simulink model "PPT_sim"  (R2023b)
settings: Solver=VariableStepAuto  StartTime=0.0  StopTime=Tstop  FixedStep=1e-9  RelTol=1e-3
values from neighbouring files (symbols this model uses):
  F_constant = (0.5 * Lpe)    (= 1.88495559215e-06)    [Electrical_model.m]
  Lpe = (mu_o/(4*pi))*log(r_o/r_i)    [Electrical_model.m]
  Re = 5e-3    (= 0.005)    [Electrical_model.m]
  Rp = 15e-3    (= 0.015)    [Electrical_model.m]
  Rpe = 5e-3    (= 0.005)    [Electrical_model.m]
libraries: fl_lib x8, nesl_utility x6, ee_lib x3
settings Model: Creator=georges  LastModifiedBy=georges

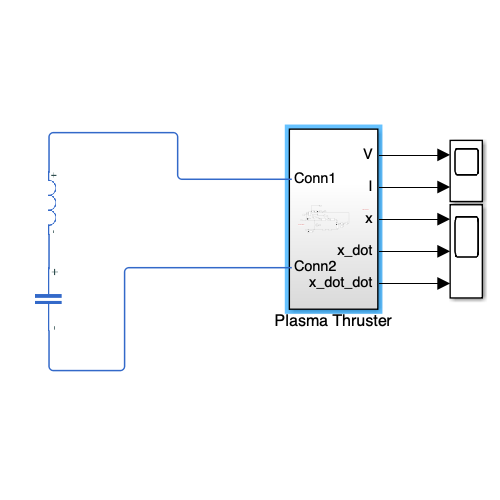
[thumbnail: Simulink's stored preview of the top-level diagram]
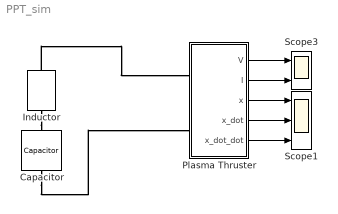
== system PPT_sim ==
  Capacitor : fl_lib/Electrical/Electrical Elements/Capacitor  c=C F  r=0 Ohm  g=0 1/Ohm  i_specify=off  i_priority=None  i=0 A  i_nominal_specify=off  i_nominal_unit=A  i_nominal_value=1  v_specify=off  v_priority=None  v=0 V  v_nominal_specify=off  v_nominal_unit=V  v_nominal_value=1  vc_specify=on  vc_priority=High  vc=V_o V  vc_nominal_specify=off  vc_nominal_unit=V  vc_nominal_value=1
  Inductor : fl_lib/Electrical/Electrical Elements/Inductor  l=C_l H  r=C_r Ohm  g=1e-9 1/Ohm  i_specify=off  i_priority=None  i=0 A  i_nominal_specify=off  i_nominal_unit=A  i_nominal_value=1  v_specify=off  v_priority=None  v=0 V  v_nominal_specify=off  v_nominal_unit=V  v_nominal_value=1  i_L_specify=off  i_L_priority=High  i_L=0 A  i_L_nominal_specify=off  i_L_nominal_unit=A  i_L_nominal_value=1
  Plasma Thruster : Subsystem
  Scope1 : Scope  NumInputPorts=3
  Scope3 : Scope  NumInputPorts=2
  wires:
  Plasma Thruster/1(V) -> Scope3/1
  Plasma Thruster/2(I) -> Scope3/2
  Plasma Thruster/3(x) -> Scope1/1
  Plasma Thruster/4(x_dot) -> Scope1/2
  Plasma Thruster/5(x_dot_dot) -> Scope1/3
  connections:
  Inductor/RConn1 -- Capacitor/LConn1
  Inductor/LConn1 -- Plasma Thruster/LConn1
  Capacitor/RConn1 -- Plasma Thruster/LConn2

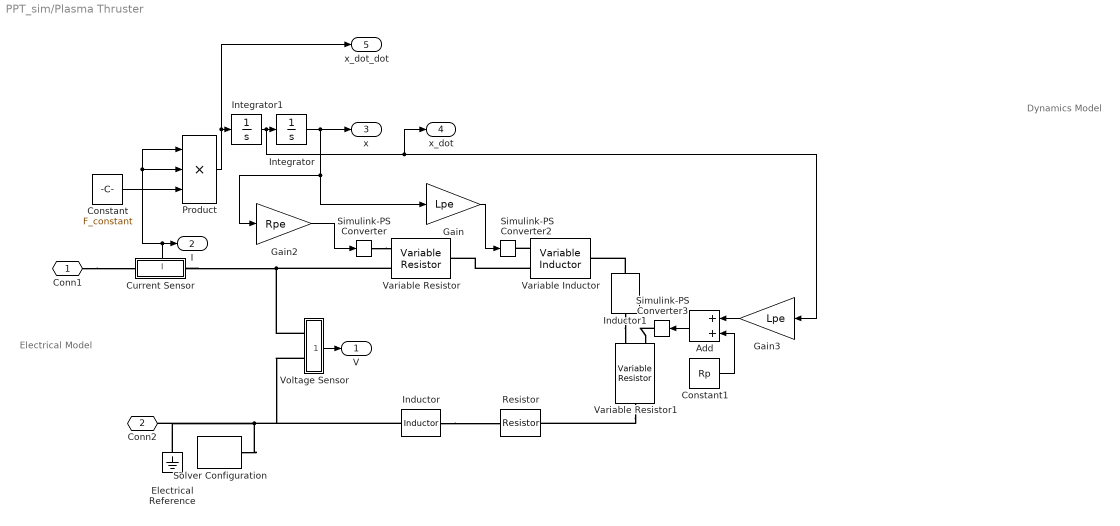
== system PPT_sim/Plasma Thruster ==
  note: Dynamics Model
  note: Electrical Model
  Add : Sum
  Constant : Constant  Value=F_constant
  Constant1 : Constant  Value=Rp
  Current Sensor : Subsystem
      settings: PortSchema="{\"entries\":[{\"content\":{\"sides\":[{\"content\":{\"connectorIds\":[\"LConn1\"]},\"type\":\"ConnectorPlacement.EquallySpacedRectSide\",\"uuid\":\"4e3d035d-d1bd-44cd-bdc3-798a8c03f7f9\"},{\"content\":{\"connectorIds\":[\"RConn1\"],\"side\":\"RIGHT\"},\"type\":\"ConnectorPlacement.EquallySpacedRectSide\",\"uuid\":\"472486ae-4f6c-481a-85ae-821eac2c32db\"},{\"content\":{\"connectorIds\":[\"Out1\"],\"side\":\"TOP\"},\"type\":\"ConnectorPlacement.EquallySpacedRectSide\",\"uuid\":\"f6d4bb52-0012-4c25-b68a-f3fc5d7680d6\"},{\"content\":{\"side\":\"BOTTOM\"},\"type\":\"ConnectorPlacement.EquallySpacedRectSide\",\"uuid\":\"a1fb2eff-50b5-40ce-849c-411f22b22d47\"}]},\"type\":\"ConnectorPlacement.EquallySpacedConnector\",\"uuid\":\"c1379bfe-a6a4-4840-8ba9-3be7ee51b238\"}],\"packageUris\":[\"http://schema.mathworks.com/mf0/Connector/R2020b\"],\"version\":\"1.0\"}"
  Electrical Reference : fl_lib/Electrical/Electrical Elements/Electrical Reference
  Gain : Gain  Gain=Lpe
  Gain2 : Gain  Gain=Rpe
  Gain3 : Gain  Gain=Lpe
  Inductor : ee_lib/Passive/Inductor  l=Le H  enable_L_tol=ee.enum.toleranceApplication.none  L_tol=20  tol_distribution=ee.enum.toleranceDistribution.uniform  nSigma=4  r=0 Ohm  g=0 1/Ohm  enable_operating_limits=ee.enum.enable.no  operating_limit_action=ee.enum.passive.reportOpLim.warn  max_working_current=1 A  power_rating=1 W  enable_faults=ee.enum.enable.no  fault_action=simscape.enum.assert.action.none  lambdaPercent=50  k_faulted=0.9999  turnsShort=ee.enum.passive.inductor.turnsShortOption.no  openCct=ee.enum.enable.no  groundShort=ee.enum.passive.inductor.groundShortOption.no  groundShortG=0 1/Ohm  tau_fault=1e-3 s  fault_trigger=ee.enum.faults.faultTrigger.temporal  t_fault=1 s  max_permissible_voltage=100 V  n_fail_on_voltage=1  max_permissible_current=1 A  t_fail_on_current=1 s  i_L_specify=off  i_L_priority=High  i_L=0 A  i_L_nominal_specify=off  i_L_nominal_unit=A  i_L_nominal_value=1
  Inductor1 : ee_lib/Passive/Inductor  l=Lp H  enable_L_tol=ee.enum.toleranceApplication.none  L_tol=20  tol_distribution=ee.enum.toleranceDistribution.uniform  nSigma=4  r=0 Ohm  g=0 1/Ohm  enable_operating_limits=ee.enum.enable.no  operating_limit_action=ee.enum.passive.reportOpLim.warn  max_working_current=1 A  power_rating=1 W  enable_faults=ee.enum.enable.no  fault_action=simscape.enum.assert.action.none  lambdaPercent=50  k_faulted=0.9999  turnsShort=ee.enum.passive.inductor.turnsShortOption.no  openCct=ee.enum.enable.no  groundShort=ee.enum.passive.inductor.groundShortOption.no  groundShortG=0 1/Ohm  tau_fault=1e-3 s  fault_trigger=ee.enum.faults.faultTrigger.temporal  t_fault=1 s  max_permissible_voltage=100 V  n_fail_on_voltage=1  max_permissible_current=1 A  t_fail_on_current=1 s  i_L_specify=off  i_L_priority=High  i_L=0 A  i_L_nominal_specify=off  i_L_nominal_unit=A  i_L_nominal_value=1
  Integrator : Integrator
  Integrator1 : Integrator
  Product : Product  Inputs=3
  Resistor : fl_lib/Electrical/Electrical Elements/Resistor  R=Re Ohm  i_specify=off  i_priority=None  i=0 A  i_nominal_specify=off  i_nominal_unit=A  i_nominal_value=1  v_specify=off  v_priority=None  v=0 V  v_nominal_specify=off  v_nominal_unit=V  v_nominal_value=1
  Simulink-PS Converter : nesl_utility/Simulink-PS Converter  PhysicalDomain=network_engine_domain  SubClassName=ps_input  LeftPortType=input  RightPortType=output  PseudoPeriodic=off  Frequencies=[]  NoiseDistribution=none  NoiseParameters=[]  Unit=1  AffineConversion=off  FilteringAndDerivatives=provide  SimscapeFilterOrder=1  InputFilterTimeConstant=0.001  UdotUserProvided=0
  Simulink-PS Converter2 : nesl_utility/Simulink-PS Converter  PhysicalDomain=network_engine_domain  SubClassName=ps_input  LeftPortType=input  RightPortType=output  PseudoPeriodic=off  Frequencies=[]  NoiseDistribution=none  NoiseParameters=[]  Unit=1  AffineConversion=off  FilteringAndDerivatives=provide  SimscapeFilterOrder=1  InputFilterTimeConstant=0.001  UdotUserProvided=0
  Simulink-PS Converter3 : nesl_utility/Simulink-PS Converter  PhysicalDomain=network_engine_domain  SubClassName=ps_input  LeftPortType=input  RightPortType=output  PseudoPeriodic=off  Frequencies=[]  NoiseDistribution=none  NoiseParameters=[]  Unit=1  AffineConversion=off  FilteringAndDerivatives=provide  SimscapeFilterOrder=1  InputFilterTimeConstant=0.001  UdotUserProvided=0
  Solver Configuration : nesl_utility/Solver Configuration  PhysicalDomain=network_engine_domain  SubClassName=solver  LeftPortType=input  RightPortType=generic  Tones=[]  Harmonics=[]  SimulateNoise=off  Profile=off  UseLocalSampling=off  EnableSwitchedLinearOptims=on  FrequencyDomain=off  UseCCode=off  RelTol=0.001  AbsTol=0.001  MinStep=1e-09  ToWorkspace=off  RevertToSquareIcSolve=off  NumHomotopyIterations=100  PhasorMode=off  PhasorModeNumHarmonics=1  ConsistencySolver=NEWTON_XTOL_AFTER_FTOL  IndexReductionMethod=DerivativeReplacement  DoDC=off  ResidualTolerance=1e-09  ConsistencyTolSource=GLOBAL  ConsistencyAbsTol=0.001  ConsistencyRelTol=0.001  ConsistencyTolFactor=0.001  UseLocalSolver=off  LocalSolverChoice=NE_BACKWARD_EULER_ADVANCER  ResolveIndetEquations=on  FunctionEvalNumThread=1  LocalSolverSampleTime=0.001  DoFixedCost=off  MaxNonlinIter=3  MaxModeIter=2  ComputeImpulses=off  ImpulseIterations=2  LinearAlgebra=auto  LinearAlgebraNumThread=0  EquationFormulation=NE_TIME_EF  DelaysMemoryBudget=1024  AutomaticFiltering=on  FilteringTimeConstant=0.001  PartitionStorageMethod=AS_NEEDED  PartitionMemoryBudget=1024  PartitionMethod=ROBUST  MultibodyUseLocalSolver=off  MultibodyLocalSolverChoice=ODE1  MultibodyLocalSolverSampleTime=0.001
  Variable Inductor : ee_lib/Passive/Variable Inductor  prm=2  Lmin=Lpe nH  g=0 1/Ohm  i0=0 A  phi0=0 Wb
      settings: InternalSimscapePortConfiguration="{\"Bottom\":[],\"Left\":[{\"id\":\"L\",\"label\":\"L\",\"type\":\"input\"},{\"id\":\"p\",\"label\":\"+\",\"type\":\"foundation.electrical.electrical\"}],\"Right\":[{\"id\":\"n\",\"label\":\"-\",\"type\":\"foundation.electrical.electrical\"}],\"Top\":[]}"
  Variable Resistor : fl_lib/Electrical/Electrical Elements/Variable Resistor  Rmin=Rpe mOhm  thermalEnable=false  thermal_mass=1 J/K  i_specify=off  i_priority=None  i=0 A  i_nominal_specify=off  i_nominal_unit=A  i_nominal_value=1  v_specify=off  v_priority=None  v=0 V  v_nominal_specify=off  v_nominal_unit=V  v_nominal_value=1  T_specify=off  T_priority=None  T=300 K  T_nominal_specify=off  T_nominal_unit=K  T_nominal_value=1
  Variable Resistor1 : fl_lib/Electrical/Electrical Elements/Variable Resistor  Rmin=Rp mOhm  thermalEnable=false  thermal_mass=1 J/K  i_specify=off  i_priority=None  i=0 A  i_nominal_specify=off  i_nominal_unit=A  i_nominal_value=1  v_specify=off  v_priority=None  v=0 V  v_nominal_specify=off  v_nominal_unit=V  v_nominal_value=1  T_specify=off  T_priority=None  T=300 K  T_nominal_specify=off  T_nominal_unit=K  T_nominal_value=1
  Voltage Sensor : Subsystem
  Conn1 : PMIOPort  Side=Left
  Conn2 : PMIOPort  Port=2  Side=Left
  V : Outport
  I : Outport  Port=2
  x : Outport  Port=3
  x_dot : Outport  Port=4
  x_dot_dot : Outport  Port=5
  wires:
  Gain/1 -> Simulink-PS Converter2/1
  Voltage Sensor/1(V) -> V/1
  Current Sensor/1(I) -> Product/1, Product/2, I/1
  Constant/1 -> Product/3
  Product/1 -> x_dot_dot/1, Integrator1/1
  Integrator/1 -> Gain/1, Gain2/1, x/1
  Add/1 -> Simulink-PS Converter3/1
  Constant1/1 -> Add/2
  Integrator1/1 -> x_dot/1, Gain3/1, Integrator/1
  Gain3/1 -> Add/1
  Gain2/1 -> Simulink-PS Converter/1
  connections:
  Solver Configuration/RConn1 -- Inductor/RConn1 -- Voltage Sensor/LConn2 -- Electrical Reference/LConn1 -- Conn2/RConn1
  Variable Inductor/LConn1 -- Simulink-PS Converter2/RConn1
  Variable Inductor/LConn2 -- Variable Resistor/RConn1
  Inductor1/RConn1 -- Variable Resistor1/LConn2
  Inductor1/LConn1 -- Variable Inductor/RConn1
  Variable Resistor1/RConn1 -- Resistor/LConn1
  Current Sensor/RConn1 -- Voltage Sensor/LConn1 -- Variable Resistor/LConn2
  Conn1/RConn1 -- Current Sensor/LConn1
  Simulink-PS Converter3/RConn1 -- Variable Resistor1/LConn1
  Inductor/LConn1 -- Resistor/RConn1
  Simulink-PS Converter/RConn1 -- Variable Resistor/LConn1

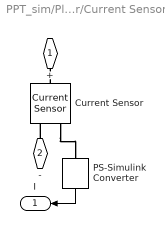
== system PPT_sim/Plasma Thruster/Current Sensor ==
  Current Sensor : fl_lib/Electrical/Electrical Sensors/Current Sensor
  PS-Simulink Converter : nesl_utility/PS-Simulink Converter  PhysicalDomain=network_engine_domain  SubClassName=ps_output  LeftPortType=input  RightPortType=output  PseudoPeriodic=off  Frequencies=[]  VectorFormat=1-D array  Unit=1  AffineConversion=off
  + : PMIOPort  Side=Left
  - : PMIOPort  Port=2  Side=Right
  I : Outport  VectorParamsAs1DForOutWhenUnconnected=off
  wires:
  PS-Simulink Converter/1 -> I/1
  connections:
  Current Sensor/LConn1 -- +/RConn1
  -/RConn1 -- Current Sensor/RConn2
  Current Sensor/RConn1 -- PS-Simulink Converter/LConn1

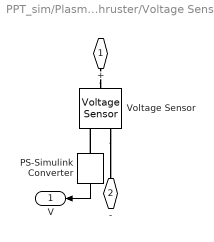
== system PPT_sim/Plasma Thruster/Voltage Sensor ==
  PS-Simulink Converter : nesl_utility/PS-Simulink Converter  PhysicalDomain=network_engine_domain  SubClassName=ps_output  LeftPortType=input  RightPortType=output  PseudoPeriodic=off  Frequencies=[]  VectorFormat=1-D array  Unit=1  AffineConversion=off
  Voltage Sensor : fl_lib/Electrical/Electrical Sensors/Voltage Sensor
  + : PMIOPort  Side=Left
  - : PMIOPort  Port=2  Side=Left
  V : Outport  VectorParamsAs1DForOutWhenUnconnected=off
  wires:
  PS-Simulink Converter/1 -> V/1
  connections:
  PS-Simulink Converter/LConn1 -- Voltage Sensor/RConn1
  Voltage Sensor/RConn2 -- -/RConn1
  +/RConn1 -- Voltage Sensor/LConn1
